simulink model "eVTOL_HIL"  (R2024b)
settings: Solver=FixedStepAuto  StartTime=0.0  StopTime=inf  FixedStep=SAMPLE_TIME  RelTol=1e-3
values from neighbouring files (symbols this model uses):
  aDl =     [initdata.mat]
  aDr =     [initdata.mat]
  aDyn =     [initdata.mat]
  aLat =     [initdata.mat]
  aLon =     [initdata.mat]
  D = Prop.D    [EOM_dt_MC.m]    (also in EOM_get_alf_dt_de_prop_evtol.m = CD * QS)
  General = init_layoutdata    [EOM_dt_MC.m]    (also in build_optimized_CA.m; initdata.mat = ; initdata_HIL_eVTOL.m)
  mass = Con(3)    [EOM_get_alf_dt_de_prop_evtol.m]    (also in initdata.mat = 2255.54; initdata_HIL_eVTOL.m = 7)
  Motor = init_motor_evtol    [EOM_dt_MC.m]    (also in initdata.mat = []; initdata_HIL_eVTOL.m)
  Prop = init_propeller_evtol_new    [EOM_dt_MC.m]    (also in initdata_HIL_eVTOL.m)
  SAMPLE_TIME = 0.01    [initdata_HIL_eVTOL.m]
undefined symbols (not defined in the file or in its folder): aDa, aDe, asbhl20env, Environment, InitData, magnitude
libraries: simulink_extras x16, vrlib x8, matrix_library x6, sharedutil x6, aerolibwindfilters x4, sharedtransform x4, aerolibfltsims x3, instrumentseriallib x3, uavmavlinklib x3, aerolibasang x3, aerolibobsolete x2, aerolibanimutils x1
(part 1 of 4)
settings Model: SimulationMode=accelerator  Creator=Administrator  LastModifiedBy=ZDB
settings DebuggingCC: UnderspecifiedInitializationDetection=Classic  MergeDetectMultiDrivingBlocksExec=none
settings ModelReferenceCC: PropagateSignalLabelsOutOfModel=off

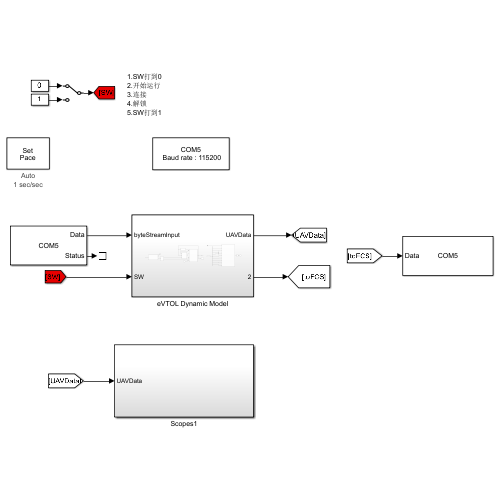
[thumbnail: Simulink's stored preview of the top-level diagram]
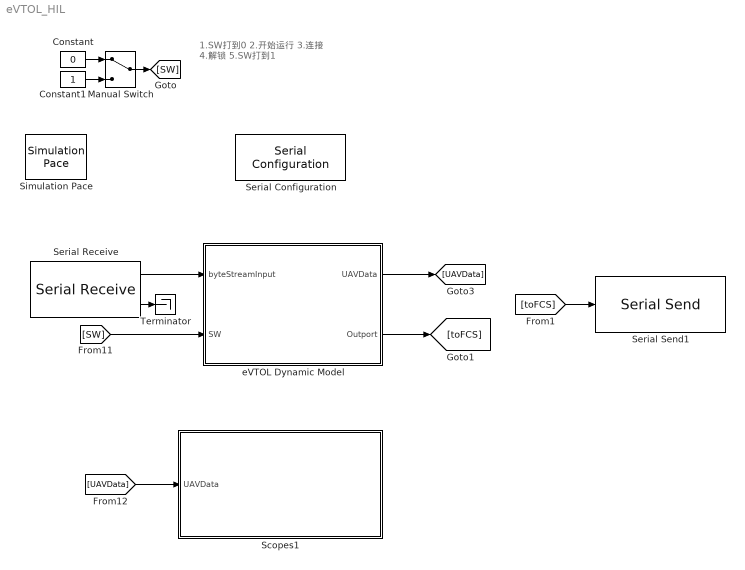
== system eVTOL_HIL ==
  note: 1.SW打到0
      | 2.开始运行
      | 3.连接
      | 4.解锁
      | 5.SW打到1
  Constant : Constant  Value=0
  Constant1 : Constant
  Manual Switch : ManualSwitch
  Scopes1 : Subsystem
  Serial Configuration : instrumentseriallib/Serial Configuration  Priority=-200000  PortSel=COM5  Port=COM5  ComPort=COM5  BaudRate=115200  DataBits=8  Parity=none  StopBits=1  ByteOrder=little-endian  FlowControl=none  Timeout=10  SimulateUsing=Interpreted execution  BlockInModel=on  aMode=1
  Serial Receive : instrumentseriallib/Serial Receive  PortSel=COM5  Port=COM5  ComPort=COM5  DataType=uint8  SaveDataType=uint8  ToggleHeader=off  Header=[253 37]  ToggleDataSize=on  DataSize=[49]  ToggleTerminator=off  Terminator=<none>  CustomTerminator=[]  InputFormat=Column major  EnableBlockingMode=off  ActionDataUnavailable=Output last received value  ActionWhenDataUnavailable=Output last received value  CustomValue=0  SampleTime=SAMPLE_TIME  SimulateUsing=Interpreted execution  BlockInModel=on  aMode=1
  Serial Send1 : instrumentseriallib/Serial Send  Priority=1  PortSel=COM5  Port=COM5  ComPort=COM5  Header=[]  Terminator=<none>  CustomTerminator=[]  EnableBlockingMode=off  SimulateUsing=Interpreted execution  BlockInModel=on  aMode=1
  Simulation Pace : aerolibanimutils/Simulation Pace  SimulationPace=1  SleepMode=Auto  OutputPaceError=off  SampleTime=-1
  Terminator : Terminator
  eVTOL Dynamic Model : Subsystem
  wires:
  Constant/1 -> Manual Switch/1
  Manual Switch/1 -> [SW]
  Constant1/1 -> Manual Switch/2
  Serial Receive/2 -> Terminator/1
  Serial Receive/1 -> eVTOL Dynamic Model/1(byteStreamInput)
  [SW] -> eVTOL Dynamic Model/2(SW)
  eVTOL Dynamic Model/1(UAVData) -> [UAVData]
  [toFCS] -> Serial Send1/1
  eVTOL Dynamic Model/2(Outport) -> [toFCS]
  [UAVData] -> Scopes1/1(UAVData)

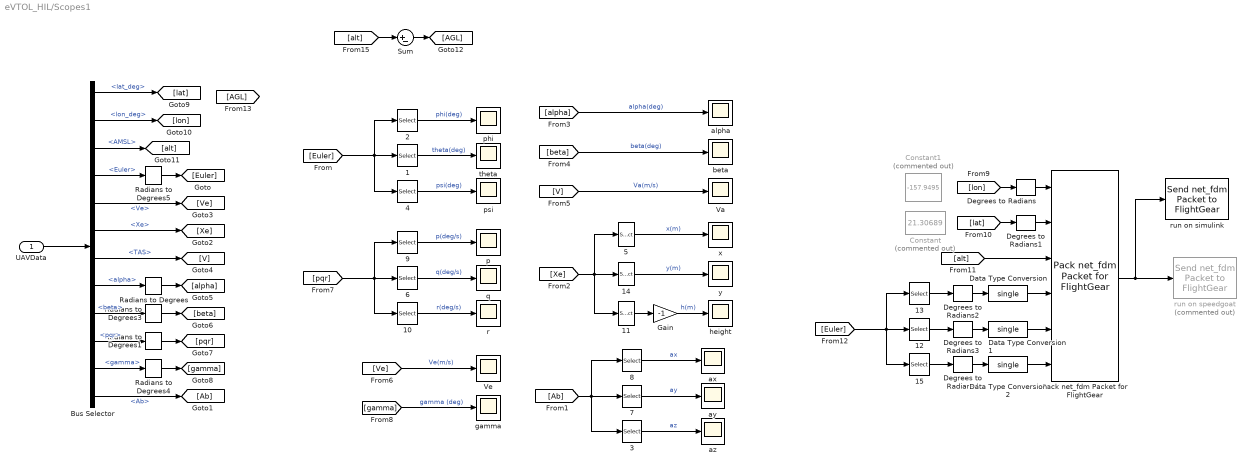
== system eVTOL_HIL/Scopes1 ==
  UAVData : Inport
  {1,6..7,12,14} (5 alike) : Selector  InputPortWidth=3  IndexOptions=Index vector (dialog)  Indices=2  OutputSizes=1
  {3..4,10..11,15} (5 alike) : Selector  InputPortWidth=3  IndexOptions=Index vector (dialog)  Indices=3  OutputSizes=1
  {2,5,8..9,13} (5 alike) : Selector  InputPortWidth=3  IndexOptions=Index vector (dialog)  Indices=1  OutputSizes=1
  Bus Selector : BusSelector  OutputSignals=lat_deg,lon_deg,AMSL,Euler,Ve,Xe,TAS,alpha,beta,pqr,gamma,Ab
  Constant : Constant  Commented=on  Value=21.30689
  Constant1 : Constant  Commented=on  Value=-157.9495
  Data Type Conversion : DataTypeConversion  OutDataTypeStr=single  SaturateOnIntegerOverflow=off  RndMeth=Floor
  Data Type Conversion1 : DataTypeConversion  OutDataTypeStr=single  SaturateOnIntegerOverflow=off  RndMeth=Floor
  Data Type Conversion2 : DataTypeConversion  OutDataTypeStr=single  SaturateOnIntegerOverflow=off  RndMeth=Floor
  Degrees to Radians{,1..4} (5 alike) : simulink_extras/Transformations/Degrees to Radians
  Gain : Gain  Gain=-1
  Pack net_fdm Packet for FlightGear : aerolibfltsims/Pack net_fdm Packet for FlightGear  FlightGearVersion=v2019.1  ShowPositionAttitudeInputs=on  ShowVelocityAccelerationInputs=off  ShowControlSurfacePositionInputs=off  ShowEngineFuelInputs=off  ShowLandingGearInputs=off  ShowEnvironmentInputs=off  SampleTime=-1  packetVersion=24
  Radians to Degrees{,1,3..5} (5 alike) : simulink_extras/Transformations/Radians to Degrees
  Sum : Sum  Inputs=|+-
  Va : Scope
  Ve : Scope
  alpha : Scope
  ax : Scope
  ay : Scope
  az : Scope
  beta : Scope
  gamma : Scope
  height : Scope
  p : Scope
  phi : Scope
  psi : Scope
  q : Scope
  r : Scope
  run on simulink : aerolibfltsims/Send net_fdm Packet to FlightGear  DestinationIpAddress=127.0.0.1  DestinationPort=5502  LocalIpPort=-1  varLen=off  SampleTime=0.01
  run on speedgoat : aerolibfltsims/Send net_fdm Packet to FlightGear  Commented=on  DestinationIpAddress=192.168.7.2  DestinationPort=5502  LocalIpPort=-1  varLen=off  SampleTime=-1
  theta : Scope
  x : Scope
  y : Scope
  wires:
  Radians to Degrees5/1 -> [Euler]
  UAVData/1 -> Bus Selector/1
  1/1 -> theta/1  "theta(deg)"
  Bus Selector/6 -> [Xe]  "<Xe>"
  2/1 -> phi/1  "phi(deg)"
  4/1 -> psi/1  "psi(deg)"
  Bus Selector/8 -> Radians to Degrees/1  "<alpha>"
  [Euler] -> 1/1, 2/1, 4/1
  Bus Selector/4 -> Radians to Degrees5/1  "<Euler>"
  [Xe] -> 5/1, 14/1, 11/1
  Bus Selector/5 -> [Ve]  "<Ve>"
  Bus Selector/7 -> [V]  "<TAS>"
  Radians to Degrees/1 -> [alpha]
  Bus Selector/9 -> Radians to Degrees3/1  "<beta>"
  Radians to Degrees3/1 -> [beta]
  [beta] -> beta/1  "beta(deg)"
  [alpha] -> alpha/1  "alpha(deg)"
  [Ve] -> Ve/1  "Ve(m/s)"
  Bus Selector/10 -> Radians to Degrees1/1  "<pqr>"
  6/1 -> q/1  "q(deg/s)"
  9/1 -> p/1  "p(deg/s)"
  10/1 -> r/1  "r(deg/s)"
  [pqr] -> 10/1, 9/1, 6/1
  Radians to Degrees1/1 -> [pqr]
  11/1 -> Gain/1
  Gain/1 -> height/1  "h(m)"
  5/1 -> x/1  "x(m)"
  Bus Selector/11 -> Radians to Degrees4/1  "<gamma>"
  Radians to Degrees4/1 -> [gamma]
  [gamma] -> gamma/1  "gamma (deg)"
  14/1 -> y/1  "y(m)"
  [V] -> Va/1  "Va(m/s)"
  Bus Selector/12 -> [Ab]  "<Ab>"
  [Ab] -> 8/1, 7/1, 3/1
  3/1 -> az/1  "az"
  8/1 -> ax/1  "ax"
  7/1 -> ay/1  "ay"
  Bus Selector/1 -> [lat]  "<lat_deg>"
  Bus Selector/2 -> [lon]  "<lon_deg>"
  Bus Selector/3 -> [alt]  "<AMSL>"
  Pack net_fdm Packet for FlightGear/1 -> run on simulink/1, run on speedgoat/1
  Degrees to Radians1/1 -> Pack net_fdm Packet for FlightGear/2
  Data Type Conversion/1 -> Pack net_fdm Packet for FlightGear/4
  Degrees to Radians/1 -> Pack net_fdm Packet for FlightGear/1
  12/1 -> Degrees to Radians3/1
  Data Type Conversion1/1 -> Pack net_fdm Packet for FlightGear/5
  13/1 -> Degrees to Radians2/1
  15/1 -> Degrees to Radians4/1
  Data Type Conversion2/1 -> Pack net_fdm Packet for FlightGear/6
  [alt] -> Pack net_fdm Packet for FlightGear/3
  Degrees to Radians2/1 -> Data Type Conversion/1
  Degrees to Radians3/1 -> Data Type Conversion1/1
  Degrees to Radians4/1 -> Data Type Conversion2/1
  [lon] -> Degrees to Radians/1
  [lat] -> Degrees to Radians1/1
  [Euler] -> 15/1, 13/1, 12/1
  Sum/1 -> [AGL]
  [alt] -> Sum/1

== system eVTOL_HIL/eVTOL Dynamic Model ==
  byteStreamInput : Inport
  SW : Inport  Port=2
  Bus Selector : BusSelector  OutputSignals=DCM_be,pqr,lat_deg,lon_deg,AMSL,Ve,Ab,EAS,TAS
  Clock1 : Clock
  Energy & Power : Subsystem
  Environment : Subsystem  AncestorBlock=asbhl20env/Environment  TreatAsAtomicUnit=on
      settings: LibrarySourceBlock=asbhl20env/Environment
  MAVLink Deserializer1 : uavmavlinklib/MAVLink Deserializer  dialectSource=Select from standard MAVLink dialects  dialect=common.xml  dialectCustom=common.xml  version=2  messageType=SERVO_OUTPUT_RAW  inputDataLength=off  SystemIDFilter=off  systemID=1  ComponentIDFilter=off  componentID=1  queueMsg=off  queueMsgSize=50  dropNum=off
  Mux : Mux  Inputs=2
  Rate Transition : RateTransition  OutPortSampleTime=0.01
  Scope1 : Scope
  airframe : Subsystem
  hil_state_quaternion_pack1 : Subsystem
  信号处理 : Subsystem
  UAVData : Outport
  Outport : Outport  Port=2
  wires:
  MAVLink Deserializer1/1 -> Scope1/1  "status"
  byteStreamInput/1 -> MAVLink Deserializer1/1
  MAVLink Deserializer1/2 -> 信号处理/1(Msg)
  SW/1 -> airframe/4(SW)
  信号处理/2(Act_surface) -> airframe/3(Act_surface)
  Energy & Power/1(PropData) -> airframe/2(prop)
  Environment/1(Envm) -> Energy & Power/1(EnvData), airframe/1(EnvmData)
  信号处理/1(Act_T) -> Energy & Power/3(Act_T)
  Bus Selector/9 -> hil_state_quaternion_pack1/9(TAS)  "<TAS>"
  Rate Transition/1 -> Outport/1
  Bus Selector/4 -> Mux/2  "<lon_deg>"
  Bus Selector/5 -> hil_state_quaternion_pack1/5(amsl)  "<AMSL>"
  Bus Selector/6 -> hil_state_quaternion_pack1/6(Ve)  "<Ve>"
  Bus Selector/3 -> Mux/1  "<lat_deg>"
  Clock1/1 -> hil_state_quaternion_pack1/1(time_s)  "time_s"
  Bus Selector/7 -> hil_state_quaternion_pack1/7(ab)  "<Ab>"
  Bus Selector/1 -> hil_state_quaternion_pack1/2(DCM_be)  "<DCM_be>"
  Bus Selector/8 -> hil_state_quaternion_pack1/8(EAS)  "<EAS>"
  Mux/1 -> hil_state_quaternion_pack1/4(latlon_deg)
  hil_state_quaternion_pack1/1(Data to px4) -> Rate Transition/1
  [UAVData] -> Bus Selector/1
  Bus Selector/2 -> hil_state_quaternion_pack1/3(body_rate)  "<pqr>"
  airframe/1(UAVData) -> [UAVData], UAVData/1, Environment/1(plane), Energy & Power/2(UAVData)

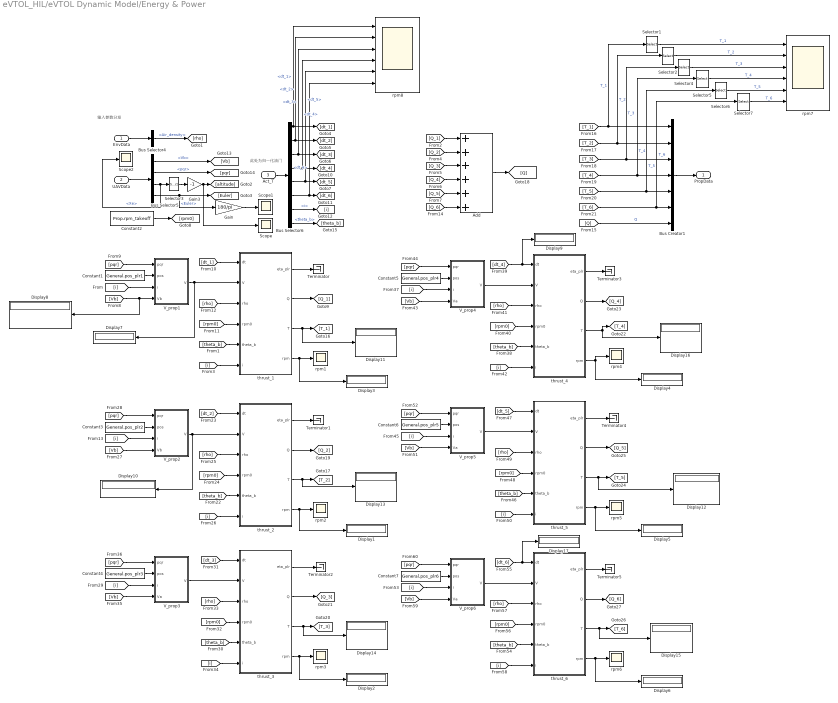
== system eVTOL_HIL/eVTOL Dynamic Model/Energy & Power ==
  note: 此处为归一化油门
  note: 输入参数分发
  EnvData : Inport
  UAVData : Inport  Port=2
  Act_T : Inport  Port=3
  Add : Sum  Inputs=++++++
  Bus Creator1 : BusCreator  Inputs=7
  Bus Selector4 : BusSelector  OutputSignals=Air_density
  Bus Selector5 : BusSelector  OutputSignals=Vb,pqr,Xe,Euler
  Bus Selector6 : BusSelector  OutputSignals=dt_1,dt_2,dt_3,dt_4,dt_5,dt_6,i,theta_b
  Constant1 : Constant  Value=General.pos_plr1
  Constant2 : Constant  Value=Prop.rpm_takeoff
  Constant3 : Constant  Value=General.pos_plr2
  Constant4 : Constant  Value=General.pos_plr3
  Constant5 : Constant  Value=General.pos_plr4
  Constant6 : Constant  Value=General.pos_plr5
  Constant7 : Constant  Value=General.pos_plr6
  Display{1..17} (17 alike) : Display
  Gain : Gain  Gain=180/pi
  Gain3 : Gain  Gain=-1
  Scope : Scope
  Scope1 : Scope
  Scope2 : Scope
  Selector{1..7} (7 alike) : Selector  InputPortWidth=3  IndexOptions=Index vector (dialog)  Indices=3  OutputSizes=1
  Terminator{,1..5} (6 alike) : Terminator
  V_prop1 : Subsystem
  V_prop2 : Subsystem
  V_prop3 : Subsystem
  V_prop4 : Subsystem
  V_prop5 : Subsystem
  V_prop6 : Subsystem
  rpm{1..6} (6 alike) : Scope
  rpm7 : Scope  NumInputPorts=6
  rpm8 : Scope  NumInputPorts=6
  thrust_1 : Subsystem
  thrust_2 : Subsystem
  thrust_3 : Subsystem
  thrust_4 : Subsystem
  thrust_5 : Subsystem
  thrust_6 : Subsystem
  PropData : Outport  VectorParamsAs1DForOutWhenUnconnected=off
  wires:
  Act_T/1 -> Bus Selector6/1
  [dt_1] -> thrust_1/1(dt)
  thrust_1/4(rpm) -> Display3/1, rpm1/1
  Constant1/1 -> V_prop1/2(pos)
  [rho] -> thrust_1/3(rho)
  [rpm0] -> thrust_1/4(rpm0)
  thrust_1/1(eta_plr) -> Terminator/1
  [pqr] -> V_prop1/1(pqr)
  [Vb] -> Display8/1, V_prop1/4(Vb)
  EnvData/1 -> Bus Selector4/1
  Bus Selector4/1 -> [rho]  "<Air_density>"
  Bus Selector5/2 -> [pqr]  "<pqr>"
  Selector3/1 -> Gain3/1
  UAVData/1 -> Bus Selector5/1
  Bus Selector5/4 -> Gain/1, [Euler]  "<Euler>"
  Bus Selector5/1 -> [Vb]  "<Vb>"
  Bus Selector5/3 -> Scope2/1, Selector3/1  "<Xe>"
  Bus Selector6/1 -> rpm8/1, [dt_1]  "<dt_1>"
  Bus Selector6/5 -> [dt_5], rpm8/5  "<dt_5>"
  Bus Selector6/3 -> [dt_3], rpm8/3  "<dt_3>"
  Bus Selector6/2 -> [dt_2], rpm8/2  "<dt_2>"
  V_prop1/1(V) -> thrust_1/2(V), Display7/1
  [i] -> V_prop1/3(i)
  Constant2/1 -> [rpm0]
  [theta_b] -> thrust_1/5(theta_b)
  thrust_1/2(Q) -> [Q_1]
  Bus Selector6/4 -> [dt_4], rpm8/4  "<dt_4>"
  Bus Selector6/6 -> rpm8/6, [dt_6]  "<dt_6>"
  Bus Selector6/7 -> [i]  "<i>"
  Bus Selector6/8 -> [theta_b]  "<theta_b>"
  [i] -> thrust_1/6(i)
  thrust_1/3(T) -> Display11/1, [T_1]
  [Q_1] -> Add/1
  [Q_6] -> Add/6
  [Q_5] -> Add/5
  [Q_4] -> Add/4
  [Q_3] -> Add/3
  [Q_2] -> Add/2
  Add/1 -> [Q]
  [Q] -> Bus Creator1/7  "Q"
  [T_1] -> Selector1/1, Bus Creator1/1  "T_1"
  [T_2] -> Selector2/1, Bus Creator1/2  "T_2"
  [T_3] -> Bus Creator1/3, Selector4/1  "T_3"
  [T_4] -> Bus Creator1/4, Selector5/1  "T_4"
  [T_5] -> Bus Creator1/5, Selector6/1  "T_5"
  [T_6] -> Bus Creator1/6, Selector7/1  "T_6"
  Bus Creator1/1 -> PropData/1
  [theta_b] -> thrust_2/5(theta_b)
  Constant3/1 -> V_prop2/2(pos)
  [dt_2] -> thrust_2/1(dt)
  V_prop2/1(V) -> Display10/1, thrust_2/2(V)
  thrust_2/2(Q) -> [Q_2]
  thrust_2/1(eta_plr) -> Terminator1/1
  [i] -> V_prop2/3(i)
  thrust_2/3(T) -> [T_2], Display13/1
  [rpm0] -> thrust_2/4(rpm0)
  [Vb] -> V_prop2/4(Vb)
  [pqr] -> V_prop2/1(pqr)
  [i] -> thrust_2/6(i)
  thrust_2/4(rpm) -> rpm2/1, Display1/1
  [rho] -> thrust_2/3(rho)
  [rho] -> thrust_3/3(rho)
  [pqr] -> V_prop3/1(pqr)
  [Vb] -> V_prop3/4(Va)
  [i] -> V_prop3/3(i)
  thrust_3/2(Q) -> [Q_3]
  V_prop3/1(V) -> thrust_3/2(V)
  [rpm0] -> thrust_3/4(rpm0)
  [dt_3] -> thrust_3/1(dt)
  thrust_3/4(rpm) -> Display2/1, rpm3/1
  [theta_b] -> thrust_3/5(theta_b)
  Constant4/1 -> V_prop3/2(pos)
  thrust_3/1(eta_plr) -> Terminator2/1
  [i] -> thrust_3/6(i)
  thrust_3/3(T) -> Display14/1, [T_3]
  [i] -> thrust_4/6(i)
  [theta_b] -> thrust_4/5(theta_b)
  Constant5/1 -> V_prop4/2(pos)
  thrust_4/1(eta_plr) -> Terminator3/1
  thrust_4/3(T) -> [T_4], Display16/1
  [dt_4] -> Display9/1, thrust_4/1(dt)
  V_prop4/1(V) -> thrust_4/2(V)
  [rpm0] -> thrust_4/4(rpm0)
  [i] -> V_prop4/3(i)
  thrust_4/4(rpm) -> rpm4/1, Display4/1
  [Vb] -> V_prop4/4(Va)
  [pqr] -> V_prop4/1(pqr)
  [rho] -> thrust_4/3(rho)
  thrust_4/2(Q) -> [Q_4]
  thrust_5/2(Q) -> [Q_5]
  thrust_5/3(T) -> Display12/1, [T_5]
  [rho] -> thrust_5/3(rho)
  [pqr] -> V_prop5/1(pqr)
  [rpm0] -> thrust_5/4(rpm0)
  Constant6/1 -> V_prop5/2(pos)
  thrust_5/1(eta_plr) -> Terminator4/1
  [dt_5] -> thrust_5/1(dt)
  thrust_5/4(rpm) -> Display5/1, rpm5/1
  [i] -> V_prop5/3(i)
  V_prop5/1(V) -> thrust_5/2(V)
  [i] -> thrust_5/6(i)
  [theta_b] -> thrust_5/5(theta_b)
  [Vb] -> V_prop5/4(Va)
  [i] -> V_prop6/3(i)
  [Vb] -> V_prop6/4(Va)
  thrust_6/1(eta_plr) -> Terminator5/1
  V_prop6/1(V) -> thrust_6/2(V)
  [dt_6] -> Display17/1, thrust_6/1(dt)
  [theta_b] -> thrust_6/5(theta_b)
  thrust_6/2(Q) -> [Q_6]
  thrust_6/3(T) -> Display15/1, [T_6]
  Constant7/1 -> V_prop6/2(pos)
  [rho] -> thrust_6/3(rho)
  thrust_6/4(rpm) -> Display6/1, rpm6/1
  [pqr] -> V_prop6/1(pqr)
  [rpm0] -> thrust_6/4(rpm0)
  [i] -> thrust_6/6(i)
  Selector1/1 -> rpm7/1  "T_1"
  Selector2/1 -> rpm7/2  "T_2"
  Selector4/1 -> rpm7/3  "T_3"
  Selector5/1 -> rpm7/4  "T_4"
  Selector6/1 -> rpm7/5  "T_5"
  Selector7/1 -> rpm7/6  "T_6"
  Gain3/1 -> Scope/1, [altitude]
  Gain/1 -> Scope1/1

== system eVTOL_HIL/eVTOL Dynamic Model/Environment ==
  plane : Inport
  Bus Creator : BusCreator  Inputs=8
  Bus Selector : BusSelector  OutputSignals=Xe,Ve,DCM_be
  COESA Atmosphere Model : aerolibatmos2/COESA Atmosphere Model  units=Metric (MKS)  spec=1976 COESA-extended U.S. Standard Atmosphere  model=Profile  profile_var=High temperature  profile_percent=1%  profile_alt=5 km (16404 ft)  envelope_var=High temperature  envelope_percent=1%  action=Warning
  Height : Selector  InputPortWidth=3  IndexOptions=Index vector (dialog)  Indices=[3]  OutputSizes=1
  Latitude : Constant  Value=40
  Terrain : Subsystem
  WGS84 Gravity Model : aerolibobsolete/WGS84 Gravity Model  model=WGS84 Taylor Series  units=Metric (MKS)  no_atmos=on  precessing=on  month=February  day=1  year=2000  no_centrifugal=on  action=None
  Wind Models : Subsystem
  x : Selector  InputPortWidth=3  IndexOptions=Index vector (dialog)  Indices=1  OutputSizes=1
  z-->h : Abs
  Envm : Outport  InitialOutput=0  VectorParamsAs1DForOutWhenUnconnected=off
  wires:
  Bus Selector/1 -> x/1, Terrain/1(Xe), Height/1  "<Xe>"
  Bus Selector/3 -> Wind Models/4(DCM)  "<DCM_be>"
  Wind Models/1(ug,vg,wg1) -> Bus Creator/2  "WindVelocity"
  Height/1 -> z-->h/1
  Latitude/1 -> WGS84 Gravity Model/2
  Wind Models/2(pg,qg,rg1) -> Bus Creator/3  "WindAngularRate"
  Bus Creator/1 -> Envm/1  "EnvmData"
  z-->h/1 -> COESA Atmosphere Model/1, WGS84 Gravity Model/1, Wind Models/3(Altitude)
  COESA Atmosphere Model/2 -> Bus Creator/5  "a"
  plane/1 -> Bus Selector/1
  COESA Atmosphere Model/3 -> Bus Creator/6  "Air_pressure"
  Bus Selector/2 -> Wind Models/2(Ve)  "<Ve>"
  COESA Atmosphere Model/4 -> Bus Creator/7  "Air_density"
  x/1 -> Wind Models/1(Xe_x)
  COESA Atmosphere Model/1 -> Bus Creator/4  "T(K)"
  Terrain/1(hground) -> Bus Creator/1  "hground"
  WGS84 Gravity Model/1 -> Bus Creator/8  "g"

== system eVTOL_HIL/eVTOL Dynamic Model/airframe ==
  EnvmData : Inport
  prop : Inport  Port=2
  Act_surface : Inport  Port=3
  SW : Inport  Port=4
  6DoF (Euler Angles)1 : aerolibobsolete/6DoF (Euler Angles)  units=Metric (MKS)  mtype=Fixed  rep=Euler Angles  xme_0=InitData.Xe  Vm_0=InitData.Vb  eul_0=InitData.Euler+[0,0,0]/57.3  pm_0=InitData.pqr  mass_0=InitData.mass0  mass_e=0.5  mass_f=2.0  inertia=Mass.Inertial  inertia_e=eye(3)  inertia_f=2*eye(3)  k_quat=1.0
  Bus Creator : BusCreator  Inputs=27
  Constant3 : Constant  Value=mass
  Flight Conditions : Subsystem  AncestorBlock=asbhl20vehicle/Vehicle/Aerodynamic/DerivedConditions
      settings: LibrarySourceBlock=asbhl20vehicle/Vehicle/Aerodynamic/DerivedConditions
  Fly : Constant
  Gain : Gain  Gain=[1,1,1]
  Gain1 : Gain  Gain=[1,1,1]
  Product : Product
  Product1 : Product
  Radians to Degrees{1..4,7..8} (6 alike) : simulink_extras/Transformations/Radians to Degrees
  Selector1 : Selector  InputPortWidth=3  IndexOptions=Index vector (dialog)  Indices=[2]  OutputSizes=1
  Selector2 : Selector  InputPortWidth=3  IndexOptions=Index vector (dialog)  Indices=[2]  OutputSizes=1
  Selector3 : Selector  InputPortWidth=3  IndexOptions=Index vector (dialog)  Indices=[1]  OutputSizes=1
  Selector4 : Selector  InputPortWidth=3  IndexOptions=Index vector (dialog)  Indices=[3]  OutputSizes=1
  Selector5 : Selector  InputPortWidth=3  IndexOptions=Index vector (dialog)  Indices=[1]  OutputSizes=1
  Selector6 : Selector  InputPortWidth=3  IndexOptions=Index vector (dialog)  Indices=[3]  OutputSizes=1
  Switch2 : Switch  Criteria=u2 > Threshold  SaturateOnIntegerOverflow=off  InputSameDT=off
  force moment : Subsystem
  fw_phi : Scope
  fw_psi : Scope
  fw_theta : Scope
  init : Constant  Value=0
  p : Scope
  q : Scope
  r : Scope
  UAVData : Outport  VectorParamsAs1DForOutWhenUnconnected=off
  wires:
  prop/1 -> force moment/3(prop)
  6DoF (Euler Angles)1/1 -> Bus Creator/1  "Ve"
  6DoF (Euler Angles)1/2 -> Bus Creator/2  "Xe"
  6DoF (Euler Angles)1/8 -> Bus Creator/8  "Ab"
  6DoF (Euler Angles)1/7 -> Bus Creator/7  "pqr_dot"
  6DoF (Euler Angles)1/5 -> Bus Creator/5  "Vb"
  Act_surface/1 -> force moment/2(Act_surface)
  Bus Creator/1 -> UAVData/1, force moment/1(PlantData), Flight Conditions/2(UAVData)  "UAVData"
  EnvmData/1 -> Flight Conditions/1(EnvData), force moment/4(EnvmData)
  6DoF (Euler Angles)1/4 -> Bus Creator/4  "DCM_be"
  Constant3/1 -> Bus Creator/23  "mass"
  force moment/1(Fb (X Y Z)) -> Gain/1
  force moment/2(M (L M N)) -> Gain1/1
  Product/1 -> 6DoF (Euler Angles)1/1
  Gain1/1 -> Product1/2
  Product1/1 -> 6DoF (Euler Angles)1/2
  Gain/1 -> Product/2
  Fly/1 -> Switch2/1
  init/1 -> Switch2/3
  Switch2/1 -> Product1/1, Product/1  "是否关闭力输出"
  SW/1 -> Switch2/2
  Flight Conditions/1(lat_deg) -> Bus Creator/9
  Flight Conditions/2(lon_deg) -> Bus Creator/10
  Flight Conditions/3(AMSL) -> Bus Creator/11
  Flight Conditions/4(gamma) -> Bus Creator/12
  Flight Conditions/5(chi) -> Bus Creator/13
  Flight Conditions/6(alphaDot) -> Bus Creator/14
  Flight Conditions/7(alpha) -> Bus Creator/15
  Flight Conditions/8(beta) -> Bus Creator/16
  Flight Conditions/9(TAS) -> Bus Creator/17
  Flight Conditions/10(pqr_air) -> Bus Creator/18
  Flight Conditions/11(Mach) -> Bus Creator/19  "mach"
  Flight Conditions/12(DynamicPressure) -> Bus Creator/20
  Flight Conditions/13(EAS) -> Bus Creator/21
  Flight Conditions/14(T(K)) -> Bus Creator/22
  Flight Conditions/15(Air_pressure) -> Bus Creator/24
  Flight Conditions/16(g) -> Bus Creator/25
  Flight Conditions/17(Vb_air) -> Bus Creator/26  "Va"
  Flight Conditions/18(Ve_Inertial) -> Bus Creator/27
  Radians to Degrees2/1 -> fw_psi/1
  Selector4/1 -> Radians to Degrees2/1
  Radians to Degrees3/1 -> fw_phi/1
  Radians to Degrees1/1 -> fw_theta/1
  6DoF (Euler Angles)1/3 -> Bus Creator/3, Selector2/1, Selector3/1, Selector4/1  "Euler"
  Selector3/1 -> Radians to Degrees3/1
  Selector2/1 -> Radians to Degrees1/1
  Radians to Degrees7/1 -> r/1
  Selector6/1 -> Radians to Degrees7/1
  Selector5/1 -> Radians to Degrees8/1
  Radians to Degrees4/1 -> q/1
  Selector1/1 -> Radians to Degrees4/1
  Radians to Degrees8/1 -> p/1
  6DoF (Euler Angles)1/6 -> Selector6/1, Selector5/1, Selector1/1, Bus Creator/6  "pqr"

== system eVTOL_HIL/eVTOL Dynamic Model/hil_state_quaternion_pack1 ==
  time_s : Inport
  DCM_be : Inport  Port=2
  body_rate : Inport  Port=3
  latlon_deg : Inport  Port=4
  amsl : Inport  Port=5
  Ve : Inport  Port=6
  ab : Inport  Port=7
  EAS : Inport  Port=8
  TAS : Inport  Port=9
  Bus Assignment : BusAssignment  AssignedSignals=signal1
  Bus Creator : BusCreator  Inputs=5  OutDataTypeStr=Bus: SL_Bus_MAVLink_HIL_STATE_QUATERNION_Packet  NonVirtualBus=on
  Bus Selector : BusSelector  OutputSignals=MsgID,SystemID,ComponentID,Sequence
  MAVLink Blank Message2 : uavmavlinklib/MAVLink Blank Message  dialectSource=Select from standard MAVLink dialects  dialect=common.xml  dialectCustom=common.xml  version=2  messageType=HIL_STATE_QUATERNION  SystemID=SYS_ID  ComponentID=COMP_ID  SampleTime=SAMPLE_TIME
  MAVLink Serializer2 : uavmavlinklib/MAVLink Serializer  dialectSource=Select from standard MAVLink dialects  dialect=common.xml  dialectCustom=common.xml  version=2  messageType=HIL_STATE_QUATERNION
  Signal Conversion : SignalConversion  ConversionOutput=Nonvirtual bus  OverrideOpt=off
  Terminator2 : Terminator
  payload_hil_state_quaternion : Subsystem
  Data to px4 : Outport
  wires:
  Signal Conversion/1 -> MAVLink Serializer2/1
  Bus Creator/1 -> Signal Conversion/1
  EAS/1 -> payload_hil_state_quaternion/8(EAS)
  ab/1 -> payload_hil_state_quaternion/7(ab)
  TAS/1 -> payload_hil_state_quaternion/9(TAS)
  Ve/1 -> payload_hil_state_quaternion/6(Ve)
  DCM_be/1 -> payload_hil_state_quaternion/2(DCM_be)
  amsl/1 -> payload_hil_state_quaternion/5(amsl)
  body_rate/1 -> payload_hil_state_quaternion/3(body_rate)
  time_s/1 -> payload_hil_state_quaternion/1(time_s)
  Bus Selector/1 -> Bus Creator/1  "<MsgID>"
  Bus Selector/2 -> Bus Creator/2  "<SystemID>"
  Bus Selector/4 -> Bus Creator/4  "<Sequence>"
  Bus Selector/3 -> Bus Creator/3  "<ComponentID>"
  payload_hil_state_quaternion/1(Payload) -> Bus Creator/5
  MAVLink Blank Message2/1 -> Bus Selector/1
  MAVLink Serializer2/1 -> Data to px4/1  "status"
  MAVLink Serializer2/2 -> Terminator2/1
  latlon_deg/1 -> payload_hil_state_quaternion/4(latlon_deg)

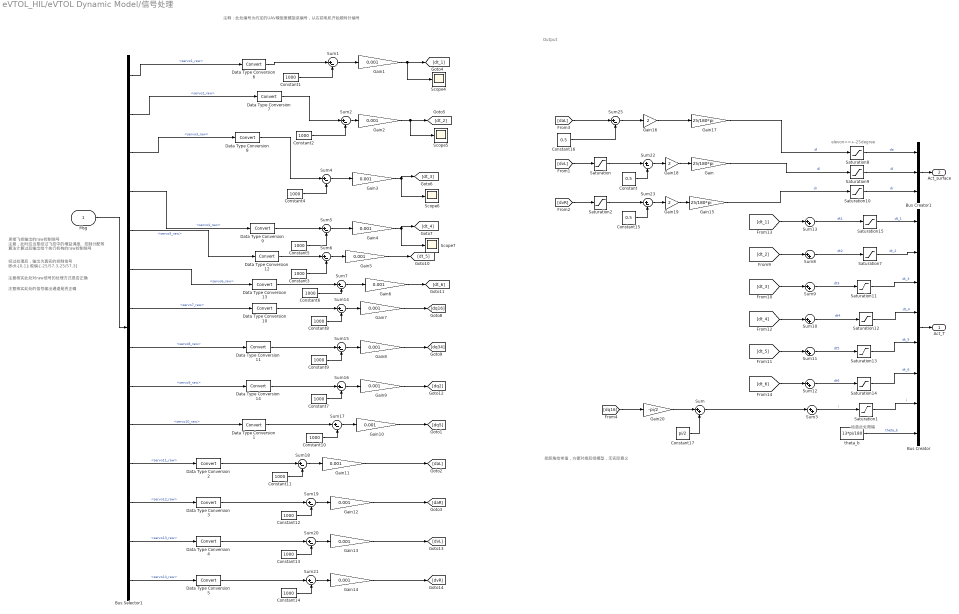
== system eVTOL_HIL/eVTOL Dynamic Model/信号处理 ==
  note: 桨距角给常值，方便对接后续模型，无实际意义
  note: 检查此处限幅
  note: 注意核实此处的信号输出通道是否正确
  note: 经过处理后，输出为真实的控制信号
      | 即dt-[0,1]; 舵偏-[-25/57.3,25/57.3]
  note: 注意核实此处对raw信号的处理方式是否正确
  note: 承接飞控输出的raw控制信号
      | 注意，此时应当是经过飞控中的增益调度、控制分配等
      | 算法计算过后输出给个执行机构的raw控制信号
  note: 注释：此处编号为约定的UAV模型里螺旋桨编号，从右前电机开始顺时针编号
  note: Output
  note: elevon==+-25degree
  Msg : Inport
  Bus Creator : BusCreator  Inputs=8
  Bus Creator1 : BusCreator  Inputs=3
  Bus Selector1 : BusSelector  OutputSignals=Payload.servo1_raw,Payload.servo2_raw,Payload.servo3_raw,Payload.servo4_raw,Payload.servo5_raw,Payload.servo6_raw,Payload.servo7_raw,Payload.servo8_raw,Payload.servo9_raw,Payload.servo10_raw,Payload.servo11_raw,Payload.servo12_raw,Payload.servo13_raw,Payload.servo14_raw
  Constant : Constant  Value=0.5
  Constant{1..14} (14 alike) : Constant  Value=1000
  Constant15 : Constant  Value=0.5
  Constant16 : Constant  Value=0.5
  Constant17 : Constant  Value=pi/2
  Data Type Conversion{1..14} (14 alike) : DataTypeConversion  SaturateOnIntegerOverflow=off  RndMeth=Floor
  Gain : Gain  Gain=25/180*pi
  Gain{1..14} (14 alike) : Gain  Gain=0.001
  Gain15 : Gain  Gain=25/180*pi
  Gain16 : Gain  Gain=2
  Gain17 : Gain  Gain=25/180*pi
  Gain18 : Gain  Gain=2
  Gain19 : Gain  Gain=2
  Gain20 : Gain  Gain=-pi/2
  Saturation{,2,7,11..15} (8 alike) : Saturate  UpperLimit=1  LowerLimit=0
  Saturation1 : Saturate  UpperLimit=90/57.3  LowerLimit=0
  Saturation10 : Saturate  UpperLimit=25/57.3  LowerLimit=-25/57.3
  Saturation8 : Saturate  UpperLimit=25/57.3  LowerLimit=-25/57.3
  Saturation9 : Saturate  UpperLimit=25/57.3  LowerLimit=-25/57.3
  Scope{4..7} (4 alike) : Scope
  Sum{,3,8..13} (8 alike) : Sum  Inputs=|++
  Sum{1..2,4..7,14..23,25} (17 alike) : Sum  Inputs=|+-
  theta_b : Constant  Value=13*pi/180
  Act_T : Outport
  Act_surface : Outport  Port=2
  wires:
  Saturation8/1 -> Bus Creator1/1  "da"
  Saturation9/1 -> Bus Creator1/2  "dl"
  Bus Creator1/1 -> Act_surface/1
  Data Type Conversion6/1 -> Sum1/1
  Gain1/1 -> [dt_1], Scope4/1
  Sum1/1 -> Gain1/1
  Constant1/1 -> Sum1/2
  Bus Selector1/1 -> Data Type Conversion6/1  "<servo1_raw>"
  Gain2/1 -> [dt_2], Scope5/1
  Constant2/1 -> Sum2/2
  Data Type Conversion7/1 -> Sum2/1
  Sum2/1 -> Gain2/1
  Bus Selector1/2 -> Data Type Conversion7/1  "<servo2_raw>"
  Gain3/1 -> [dt_3], Scope6/1
  Constant4/1 -> Sum4/2
  Data Type Conversion8/1 -> Sum4/1
  Sum4/1 -> Gain3/1
  Bus Selector1/3 -> Data Type Conversion8/1  "<servo3_raw>"
  Gain4/1 -> [dt_4], Scope7/1
  Constant5/1 -> Sum5/2
  Data Type Conversion9/1 -> Sum5/1
  Sum5/1 -> Gain4/1
  Bus Selector1/4 -> Data Type Conversion9/1  "<servo4_raw>"
  Gain7/1 -> [dq16]
  Data Type Conversion10/1 -> Sum14/1
  Gain/1 -> Saturation9/1  "dl"
  Msg/1 -> Bus Selector1/1
  Gain5/1 -> [dt_5]
  Sum6/1 -> Gain5/1
  Data Type Conversion12/1 -> Sum6/1
  Bus Selector1/5 -> Data Type Conversion12/1  "<servo5_raw>"
  Gain6/1 -> [dt_6]
  Sum7/1 -> Gain6/1
  Bus Selector1/6 -> Data Type Conversion13/1  "<servo6_raw>"
  Bus Selector1/7 -> Data Type Conversion10/1  "<servo7_raw>"
  Bus Selector1/8 -> Data Type Conversion11/1  "<servo8_raw>"
  Bus Selector1/9 -> Data Type Conversion14/1  "<servo9_raw>"
  Gain15/1 -> Saturation10/1  "dr"
  Saturation10/1 -> Bus Creator1/3  "dr"
  [dt_6] -> Sum12/1
  [dt_4] -> Sum10/1
  Saturation7/1 -> Bus Creator/2  "dt_2"
  [dt_5] -> Sum11/1
  [dt_3] -> Sum9/1
  Sum11/1 -> Saturation13/1  "dt5"
  Saturation13/1 -> Bus Creator/5  "dt_5"
  Saturation14/1 -> Bus Creator/6  "dt_6"
  Sum8/1 -> Saturation7/1  "dt2"
  Saturation15/1 -> Bus Creator/1  "dt_1"
  Sum12/1 -> Saturation14/1  "dt6"
  [dt_2] -> Sum8/1
  Sum9/1 -> Saturation11/1  "dt3"
  Sum10/1 -> Saturation12/1  "dt4"
  Sum13/1 -> Saturation15/1  "dt1"
  [dt_1] -> Sum13/1
  Saturation11/1 -> Bus Creator/3  "dt_3"
  Saturation12/1 -> Bus Creator/4  "dt_4"
  Gain10/1 -> [dq5]
  Bus Selector1/10 -> Data Type Conversion1/1  "<servo10_raw>"
  Bus Creator/1 -> Act_T/1
  Saturation1/1 -> Bus Creator/7  "i"
  Sum3/1 -> Saturation1/1  "i"
  Sum/1 -> Sum3/1
  theta_b/1 -> Bus Creator/8  "theta_b"
  Bus Selector1/11 -> Data Type Conversion2/1  "<servo11_raw>"
  Bus Selector1/12 -> Data Type Conversion3/1  "<servo12_raw>"
  Bus Selector1/13 -> Data Type Conversion4/1  "<servo13_raw>"
  Bus Selector1/14 -> Data Type Conversion5/1  "<servo14_raw>"
  Constant3/1 -> Sum6/2
  Data Type Conversion13/1 -> Sum7/1
  Constant6/1 -> Sum7/2
  Constant8/1 -> Sum14/2
  Sum14/1 -> Gain7/1
  Constant9/1 -> Sum15/2
  Sum15/1 -> Gain8/1
  Data Type Conversion11/1 -> Sum15/1
  Gain8/1 -> [dq34]
  Constant7/1 -> Sum16/2
  Sum16/1 -> Gain9/1
  Data Type Conversion14/1 -> Sum16/1
  Gain9/1 -> [dq2]
  Constant10/1 -> Sum17/2
  Sum17/1 -> Gain10/1
  Data Type Conversion1/1 -> Sum17/1
  Constant11/1 -> Sum18/2
  Sum18/1 -> Gain11/1
  Data Type Conversion2/1 -> Sum18/1
  Gain11/1 -> [daL]
  Constant12/1 -> Sum19/2
  Sum19/1 -> Gain12/1
  Data Type Conversion3/1 -> Sum19/1
  Constant13/1 -> Sum20/2
  Sum20/1 -> Gain13/1
  Data Type Conversion4/1 -> Sum20/1
  Constant14/1 -> Sum21/2
  Sum21/1 -> Gain14/1
  Data Type Conversion5/1 -> Sum21/1
  Gain14/1 -> [dvR]
  Gain13/1 -> [dvL]
  Gain12/1 -> [daR]
  Sum23/1 -> Gain19/1
  Saturation2/1 -> Sum23/1
  Sum22/1 -> Gain18/1
  Constant15/1 -> Sum23/2
  [dvL] -> Saturation/1
  Saturation/1 -> Sum22/1
  [dvR] -> Saturation2/1
  Constant/1 -> Sum22/2
  Sum25/1 -> Gain16/1
  [daL] -> Sum25/1
  Gain16/1 -> Gain17/1
  Constant16/1 -> Sum25/2
  Gain17/1 -> Saturation8/1  "dl"
  Gain18/1 -> Gain/1
  Gain19/1 -> Gain15/1
  [dq16] -> Gain20/1
  Gain20/1 -> Sum/1
  Constant17/1 -> Sum/2

== system eVTOL_HIL/eVTOL Dynamic Model/Energy & Power/V_prop1 ==
  note: 将速度矢量投影到桨轴
  pqr : Inport
  pos : Inport  Port=2
  i : Inport  Port=3
  Vb : Inport  Port=4
  Cross Product4 : matrix_library/Cross Product
  Display1 : Display
  Display2 : Display
  Display8 : Display
  Sum2 : Sum  Inputs=|++
  v_b to v_prop : Subsystem
  V : Outport
  wires:
  pos/1 -> Cross Product4/2
  pqr/1 -> Cross Product4/1
  Vb/1 -> Display2/1, Sum2/2
  i/1 -> v_b to v_prop/2(i)
  Cross Product4/1 -> Display8/1, Sum2/1
  Sum2/1 -> Display1/1, v_b to v_prop/1(V_body)
  v_b to v_prop/1(V) -> V/1

== system eVTOL_HIL/eVTOL Dynamic Model/Energy & Power/V_prop2 ==
  note: 将速度矢量投影到桨轴
  pqr : Inport
  pos : Inport  Port=2
  i : Inport  Port=3
  Vb : Inport  Port=4
  Cross Product4 : matrix_library/Cross Product
  Sum2 : Sum  Inputs=|++
  v_b to v_prop : Subsystem
  V : Outport
  wires:
  pos/1 -> Cross Product4/2
  pqr/1 -> Cross Product4/1
  Vb/1 -> Sum2/2
  i/1 -> v_b to v_prop/2(i)
  Cross Product4/1 -> Sum2/1
  Sum2/1 -> v_b to v_prop/1(V_body)
  v_b to v_prop/1(V) -> V/1

== system eVTOL_HIL/eVTOL Dynamic Model/Energy & Power/V_prop3 ==
  note: 将速度矢量投影到桨轴
  pqr : Inport
  pos : Inport  Port=2
  i : Inport  Port=3
  Va : Inport  Port=4
  Cross Product4 : matrix_library/Cross Product
  Sum2 : Sum  Inputs=|++
  v_b to v_prop : Subsystem
  V : Outport
  wires:
  pos/1 -> Cross Product4/2
  pqr/1 -> Cross Product4/1
  Va/1 -> Sum2/2
  i/1 -> v_b to v_prop/2(i)
  Cross Product4/1 -> Sum2/1
  Sum2/1 -> v_b to v_prop/1(V_body)
  v_b to v_prop/1(V) -> V/1

== system eVTOL_HIL/eVTOL Dynamic Model/Energy & Power/V_prop4 ==
  note: 将速度矢量投影到桨轴
  pqr : Inport
  pos : Inport  Port=2
  i : Inport  Port=3
  Va : Inport  Port=4
  Cross Product4 : matrix_library/Cross Product
  Sum2 : Sum  Inputs=|++
  v_b to v_prop : Subsystem
  V : Outport
  wires:
  pos/1 -> Cross Product4/2
  pqr/1 -> Cross Product4/1
  Va/1 -> Sum2/2
  i/1 -> v_b to v_prop/2(i)
  Cross Product4/1 -> Sum2/1
  Sum2/1 -> v_b to v_prop/1(V_body)
  v_b to v_prop/1(V) -> V/1

== system eVTOL_HIL/eVTOL Dynamic Model/Energy & Power/V_prop5 ==
  note: 将速度矢量投影到桨轴
  pqr : Inport
  pos : Inport  Port=2
  i : Inport  Port=3
  Va : Inport  Port=4
  Cross Product4 : matrix_library/Cross Product
  Sum2 : Sum  Inputs=|++
  v_b to v_prop : Subsystem
  V : Outport
  wires:
  pos/1 -> Cross Product4/2
  pqr/1 -> Cross Product4/1
  Va/1 -> Sum2/2
  i/1 -> v_b to v_prop/2(i)
  Cross Product4/1 -> Sum2/1
  Sum2/1 -> v_b to v_prop/1(V_body)
  v_b to v_prop/1(V) -> V/1

== system eVTOL_HIL/eVTOL Dynamic Model/Energy & Power/V_prop6 ==
  note: 将速度矢量投影到桨轴
  pqr : Inport
  pos : Inport  Port=2
  i : Inport  Port=3
  Va : Inport  Port=4
  Cross Product4 : matrix_library/Cross Product
  Sum2 : Sum  Inputs=|++
  v_b to v_prop : Subsystem
  V : Outport
  wires:
  pos/1 -> Cross Product4/2
  pqr/1 -> Cross Product4/1
  Va/1 -> Sum2/2
  i/1 -> v_b to v_prop/2(i)
  Cross Product4/1 -> Sum2/1
  Sum2/1 -> v_b to v_prop/1(V_body)
  v_b to v_prop/1(V) -> V/1

== system eVTOL_HIL/eVTOL Dynamic Model/Energy & Power/thrust_1 ==
  note: 将推力、扭矩按电机倾转角转化为向量
  note: 求桨的推力、扭矩、功率、效率
  dt : Inport
  V : Inport  Port=2
  rho : Inport  Port=3
  rpm0 : Inport  Port=4
  theta_b : Inport  Port=5
  i : Inport  Port=6
  Constant : Constant  Commented=on  Value=2.5
  Gain2 : Gain  Gain=-1
  Gain4 : Gain  Gain=pi/30
  Manual Switch : ManualSwitch  Commented=on  CurrentSetting=0
  Motor : Subsystem
  Mux1 : Mux  Inputs=2
  Mux2 : Mux  Inputs=3
  Mux3 : Mux  Inputs=2
  Mux4 : Mux  Inputs=3
  Product : Product  Inputs=*/
  "Propeller " : Subsystem
  Q_x : Fcn  Expr=-u[1]*cos(u[2])
  Q_y : Fcn  Expr=0
  Q_z : Fcn  Expr=u[1]*sin(u[2])
  Saturation : Saturate  UpperLimit=inf  LowerLimit=1
  T_x : Fcn  Expr=u[1]*cos(u[2])
  T_y : Fcn  Expr=0
  T_z : Fcn  Expr=-u[1]*sin(u[2])
  eta_plr : Outport  VectorParamsAs1DForOutWhenUnconnected=off
  Q : Outport  Port=2
  T : Outport  Port=3  VectorParamsAs1DForOutWhenUnconnected=off
  rpm : Outport  Port=4  VectorParamsAs1DForOutWhenUnconnected=off
  wires:
  Saturation/1 -> Motor/4(rpm0)
  rpm0/1 -> Saturation/1
  "Propeller "/2(T (N)) -> [T]
  dt/1 -> Motor/2(dt)
  Motor/1(rpm) -> rpm/1, Gain4/1, "Propeller "/1(rpm)
  "Propeller "/3(eta_p) -> eta_plr/1
  rho/1 -> [rho]
  "Propeller "/1(P_plr (w)) -> Motor/1(P_shaft), Product/1
  theta_b/1 -> Motor/6(theta_b), "Propeller "/4(theta_b)
  Gain4/1 -> Product/2  "omega"
  Product/1 -> Gain2/1
  T_y/1 -> Mux2/2
  Mux1/1 -> T_z/1, T_x/1, T_y/1
  T_x/1 -> Mux2/1
  i/1 -> [i]
  T_z/1 -> Mux2/3
  Mux2/1 -> T/1
  [T] -> Mux1/1
  Mux4/1 -> Q/1
  [i] -> Mux3/2
  Q_z/1 -> Mux4/3
  Q_x/1 -> Mux4/1
  Mux3/1 -> Q_z/1, Q_x/1, Q_y/1
  Q_y/1 -> Mux4/2
  [Q] -> Mux3/1
  [i] -> Mux1/2
  Gain2/1 -> [Q]
  [V] -> Motor/3(V)
  [V] -> "Propeller "/2(V)
  [rho] -> Motor/5(rho)
  [rho] -> "Propeller "/3(rho)
  Constant/1 -> Manual Switch/1
  V/1 -> [V]

== system eVTOL_HIL/eVTOL Dynamic Model/Energy & Power/thrust_2 ==
  note: 将推力、扭矩按电机倾转角转化为向量
  note: 求桨的推力、扭矩、功率、效率
  dt : Inport
  V : Inport  Port=2
  rho : Inport  Port=3
  rpm0 : Inport  Port=4
  theta_b : Inport  Port=5
  i : Inport  Port=6
  Constant : Constant  Commented=on  Value=2.5
  Gain4 : Gain  Gain=pi/30
  Manual Switch : ManualSwitch  Commented=on  CurrentSetting=0
  Motor : Subsystem
  Mux1 : Mux  Inputs=2
  Mux2 : Mux  Inputs=3
  Mux3 : Mux  Inputs=2
  Mux4 : Mux  Inputs=3
  Product : Product  Inputs=*/
  "Propeller " : Subsystem
  Q_x : Fcn  Expr=-u[1]*cos(u[2])
  Q_y : Fcn  Expr=0
  Q_z : Fcn  Expr=u[1]*sin(u[2])
  Saturation : Saturate  UpperLimit=inf  LowerLimit=1
  T_x : Fcn  Expr=u[1]*cos(u[2])
  T_y : Fcn  Expr=0
  T_z : Fcn  Expr=-u[1]*sin(u[2])
  eta_plr : Outport  VectorParamsAs1DForOutWhenUnconnected=off
  Q : Outport  Port=2
  T : Outport  Port=3  VectorParamsAs1DForOutWhenUnconnected=off
  rpm : Outport  Port=4  VectorParamsAs1DForOutWhenUnconnected=off
  wires:
  Saturation/1 -> Motor/4(rpm0)
  rpm0/1 -> Saturation/1
  "Propeller "/2(T (N)) -> [T]
  dt/1 -> Motor/2(dt)
  Motor/1(rpm) -> rpm/1, Gain4/1, "Propeller "/1(rpm)
  "Propeller "/3(eta_p) -> eta_plr/1
  rho/1 -> [rho]
  "Propeller "/1(P_plr (w)) -> Motor/1(P_shaft), Product/1
  theta_b/1 -> Motor/6(theta_b), "Propeller "/4(theta_b)
  Gain4/1 -> Product/2  "omega"
  T_y/1 -> Mux2/2
  Mux1/1 -> T_z/1, T_x/1, T_y/1
  T_x/1 -> Mux2/1
  i/1 -> [i]
  T_z/1 -> Mux2/3
  Mux2/1 -> T/1
  [T] -> Mux1/1
  Mux4/1 -> Q/1
  [i] -> Mux3/2
  Q_z/1 -> Mux4/3
  Q_x/1 -> Mux4/1
  Mux3/1 -> Q_z/1, Q_x/1, Q_y/1
  Q_y/1 -> Mux4/2
  [Q] -> Mux3/1
  [i] -> Mux1/2
  Product/1 -> [Q]
  [V] -> Motor/3(V)
  [V] -> "Propeller "/2(V)
  [rho] -> Motor/5(rho)
  [rho] -> "Propeller "/3(rho)
  Constant/1 -> Manual Switch/1
  V/1 -> [V]

== system eVTOL_HIL/eVTOL Dynamic Model/Energy & Power/thrust_3 ==
  note: 将推力、扭矩按电机倾转角转化为向量
  note: 求桨的推力、扭矩、功率、效率
  dt : Inport
  V : Inport  Port=2
  rho : Inport  Port=3
  rpm0 : Inport  Port=4
  theta_b : Inport  Port=5
  i : Inport  Port=6
  Constant : Constant  Commented=on  Value=2.5
  Gain4 : Gain  Gain=pi/30
  Manual Switch : ManualSwitch  Commented=on  CurrentSetting=0
  Motor : Subsystem
  Mux1 : Mux  Inputs=2
  Mux2 : Mux  Inputs=3
  Mux3 : Mux  Inputs=2
  Mux4 : Mux  Inputs=3
  Product : Product  Inputs=*/
  "Propeller " : Subsystem
  Q_x : Fcn  Expr=-u[1]*cos(u[2])
  Q_y : Fcn  Expr=0
  Q_z : Fcn  Expr=u[1]*sin(u[2])
  Saturation : Saturate  UpperLimit=inf  LowerLimit=1
  T_x : Fcn  Expr=u[1]*cos(u[2])
  T_y : Fcn  Expr=0
  T_z : Fcn  Expr=-u[1]*sin(u[2])
  eta_plr : Outport  VectorParamsAs1DForOutWhenUnconnected=off
  Q : Outport  Port=2
  T : Outport  Port=3  VectorParamsAs1DForOutWhenUnconnected=off
  rpm : Outport  Port=4  VectorParamsAs1DForOutWhenUnconnected=off
  wires:
  Saturation/1 -> Motor/4(rpm0)
  rpm0/1 -> Saturation/1
  "Propeller "/2(T (N)) -> [T]
  dt/1 -> Motor/2(dt)
  Motor/1(rpm) -> rpm/1, Gain4/1, "Propeller "/1(rpm)
  "Propeller "/3(eta_p) -> eta_plr/1
  rho/1 -> [rho]
  "Propeller "/1(P_plr (w)) -> Motor/1(P_shaft), Product/1
  theta_b/1 -> Motor/6(theta_b), "Propeller "/4(theta_b)
  Gain4/1 -> Product/2  "omega"
  T_y/1 -> Mux2/2
  Mux1/1 -> T_z/1, T_x/1, T_y/1
  T_x/1 -> Mux2/1
  i/1 -> [i]
  T_z/1 -> Mux2/3
  Mux2/1 -> T/1
  [T] -> Mux1/1
  Mux4/1 -> Q/1
  [i] -> Mux3/2
  Q_z/1 -> Mux4/3
  Q_x/1 -> Mux4/1
  Mux3/1 -> Q_z/1, Q_x/1, Q_y/1
  Q_y/1 -> Mux4/2
  [Q] -> Mux3/1
  [i] -> Mux1/2
  Product/1 -> [Q]
  [V] -> Motor/3(V)
  [V] -> "Propeller "/2(V)
  [rho] -> Motor/5(rho)
  [rho] -> "Propeller "/3(rho)
  Constant/1 -> Manual Switch/1
  V/1 -> [V]

== system eVTOL_HIL/eVTOL Dynamic Model/Energy & Power/thrust_4 ==
  note: 将推力、扭矩按电机倾转角转化为向量
  note: 求桨的推力、扭矩、功率、效率
  dt : Inport
  V : Inport  Port=2
  rho : Inport  Port=3
  rpm0 : Inport  Port=4
  theta_b : Inport  Port=5
  i : Inport  Port=6
  Constant : Constant  Commented=on  Value=2.5
  Gain2 : Gain  Gain=-1
  Gain4 : Gain  Gain=pi/30
  Manual Switch : ManualSwitch  Commented=on  CurrentSetting=0
  Motor : Subsystem
  Mux1 : Mux  Inputs=2
  Mux2 : Mux  Inputs=3
  Mux3 : Mux  Inputs=2
  Mux4 : Mux  Inputs=3
  Product : Product  Inputs=*/
  "Propeller " : Subsystem
  Q_x : Fcn  Expr=-u[1]*cos(u[2])
  Q_y : Fcn  Expr=0
  Q_z : Fcn  Expr=u[1]*sin(u[2])
  Saturation : Saturate  UpperLimit=inf  LowerLimit=1
  T_x : Fcn  Expr=u[1]*cos(u[2])
  T_y : Fcn  Expr=0
  T_z : Fcn  Expr=-u[1]*sin(u[2])
  eta_plr : Outport  VectorParamsAs1DForOutWhenUnconnected=off
  Q : Outport  Port=2
  T : Outport  Port=3  VectorParamsAs1DForOutWhenUnconnected=off
  rpm : Outport  Port=4  VectorParamsAs1DForOutWhenUnconnected=off
  wires:
  Saturation/1 -> Motor/4(rpm0)
  rpm0/1 -> Saturation/1
  "Propeller "/2(T (N)) -> [T]
  dt/1 -> Motor/2(dt)
  Motor/1(rpm) -> rpm/1, Gain4/1, "Propeller "/1(rpm)
  "Propeller "/3(eta_p) -> eta_plr/1
  rho/1 -> [rho]
  "Propeller "/1(P_plr (w)) -> Motor/1(P_shaft), Product/1
  theta_b/1 -> Motor/6(theta_b), "Propeller "/4(theta_b)
  Gain4/1 -> Product/2  "omega"
  T_y/1 -> Mux2/2
  Mux1/1 -> T_z/1, T_x/1, T_y/1
  T_x/1 -> Mux2/1
  i/1 -> [i]
  T_z/1 -> Mux2/3
  Mux2/1 -> T/1
  [T] -> Mux1/1
  Mux4/1 -> Q/1
  [i] -> Mux3/2
  Q_z/1 -> Mux4/3
  Q_x/1 -> Mux4/1
  Mux3/1 -> Q_z/1, Q_x/1, Q_y/1
  Q_y/1 -> Mux4/2
  [Q] -> Mux3/1
  [i] -> Mux1/2
  Product/1 -> Gain2/1
  [V] -> Motor/3(V)
  [V] -> "Propeller "/2(V)
  [rho] -> Motor/5(rho)
  [rho] -> "Propeller "/3(rho)
  Gain2/1 -> [Q]
  Constant/1 -> Manual Switch/1
  V/1 -> [V]

== system eVTOL_HIL/eVTOL Dynamic Model/Energy & Power/thrust_5 ==
  note: 将推力、扭矩按电机倾转角转化为向量
  note: 求桨的推力、扭矩、功率、效率
  dt : Inport
  V : Inport  Port=2
  rho : Inport  Port=3
  rpm0 : Inport  Port=4
  theta_b : Inport  Port=5
  i : Inport  Port=6
  Constant : Constant  Commented=on  Value=2.5
  Gain2 : Gain  Gain=-1
  Gain4 : Gain  Gain=pi/30
  Manual Switch : ManualSwitch  Commented=on  CurrentSetting=0
  Motor : Subsystem
  Mux1 : Mux  Inputs=2
  Mux2 : Mux  Inputs=3
  Mux3 : Mux  Inputs=2
  Mux4 : Mux  Inputs=3
  Product : Product  Inputs=*/
  "Propeller " : Subsystem
  Q_x : Fcn  Expr=-u[1]*cos(u[2])
  Q_y : Fcn  Expr=0
  Q_z : Fcn  Expr=u[1]*sin(u[2])
  Saturation : Saturate  UpperLimit=inf  LowerLimit=1
  T_x : Fcn  Expr=u[1]*cos(u[2])
  T_y : Fcn  Expr=0
  T_z : Fcn  Expr=-u[1]*sin(u[2])
  eta_plr : Outport  VectorParamsAs1DForOutWhenUnconnected=off
  Q : Outport  Port=2
  T : Outport  Port=3  VectorParamsAs1DForOutWhenUnconnected=off
  rpm : Outport  Port=4  VectorParamsAs1DForOutWhenUnconnected=off
  wires:
  Saturation/1 -> Motor/4(rpm0)
  rpm0/1 -> Saturation/1
  "Propeller "/2(T (N)) -> [T]
  dt/1 -> Motor/2(dt)
  Motor/1(rpm) -> rpm/1, Gain4/1, "Propeller "/1(rpm)
  "Propeller "/3(eta_p) -> eta_plr/1
  rho/1 -> [rho]
  "Propeller "/1(P_plr (w)) -> Motor/1(P_shaft), Product/1
  theta_b/1 -> Motor/6(theta_b), "Propeller "/4(theta_b)
  Gain4/1 -> Product/2  "omega"
  T_y/1 -> Mux2/2
  Mux1/1 -> T_z/1, T_x/1, T_y/1
  T_x/1 -> Mux2/1
  i/1 -> [i]
  T_z/1 -> Mux2/3
  Mux2/1 -> T/1
  [T] -> Mux1/1
  Mux4/1 -> Q/1
  [i] -> Mux3/2
  Q_z/1 -> Mux4/3
  Q_x/1 -> Mux4/1
  Mux3/1 -> Q_z/1, Q_x/1, Q_y/1
  Q_y/1 -> Mux4/2
  [Q] -> Mux3/1
  [i] -> Mux1/2
  Product/1 -> Gain2/1
  [V] -> Motor/3(V)
  [V] -> "Propeller "/2(V)
  [rho] -> Motor/5(rho)
  [rho] -> "Propeller "/3(rho)
  Gain2/1 -> [Q]
  Constant/1 -> Manual Switch/1
  V/1 -> [V]

== system eVTOL_HIL/eVTOL Dynamic Model/Energy & Power/thrust_6 ==
  note: 将推力、扭矩按电机倾转角转化为向量
  note: 求桨的推力、扭矩、功率、效率
  dt : Inport
  V : Inport  Port=2
  rho : Inport  Port=3
  rpm0 : Inport  Port=4
  theta_b : Inport  Port=5
  i : Inport  Port=6
  Constant : Constant  Commented=on  Value=2.5
  Gain4 : Gain  Gain=pi/30
  Manual Switch : ManualSwitch  Commented=on  CurrentSetting=0
  Motor : Subsystem
  Mux1 : Mux  Inputs=2
  Mux2 : Mux  Inputs=3
  Mux3 : Mux  Inputs=2
  Mux4 : Mux  Inputs=3
  Product : Product  Inputs=*/
  "Propeller " : Subsystem
  Q_x : Fcn  Expr=-u[1]*cos(u[2])
  Q_y : Fcn  Expr=0
  Q_z : Fcn  Expr=u[1]*sin(u[2])
  Saturation : Saturate  UpperLimit=inf  LowerLimit=1
  T_x : Fcn  Expr=u[1]*cos(u[2])
  T_y : Fcn  Expr=0
  T_z : Fcn  Expr=-u[1]*sin(u[2])
  eta_plr : Outport  VectorParamsAs1DForOutWhenUnconnected=off
  Q : Outport  Port=2
  T : Outport  Port=3  VectorParamsAs1DForOutWhenUnconnected=off
  rpm : Outport  Port=4  VectorParamsAs1DForOutWhenUnconnected=off
  wires:
  Saturation/1 -> Motor/4(rpm0)
  rpm0/1 -> Saturation/1
  "Propeller "/2(T (N)) -> [T]
  dt/1 -> Motor/2(dt)
  Motor/1(rpm) -> rpm/1, Gain4/1, "Propeller "/1(rpm)
  "Propeller "/3(eta_p) -> eta_plr/1
  rho/1 -> [rho]
  "Propeller "/1(P_plr (w)) -> Motor/1(P_shaft), Product/1
  theta_b/1 -> Motor/6(theta_b), "Propeller "/4(theta_b)
  Gain4/1 -> Product/2  "omega"
  T_y/1 -> Mux2/2
  Mux1/1 -> T_z/1, T_x/1, T_y/1
  T_x/1 -> Mux2/1
  i/1 -> [i]
  T_z/1 -> Mux2/3
  Mux2/1 -> T/1
  [T] -> Mux1/1
  Mux4/1 -> Q/1
  [i] -> Mux3/2
  Q_z/1 -> Mux4/3
  Q_x/1 -> Mux4/1
  Mux3/1 -> Q_z/1, Q_x/1, Q_y/1
  Q_y/1 -> Mux4/2
  [Q] -> Mux3/1
  [i] -> Mux1/2
  [V] -> Motor/3(V)
  [V] -> "Propeller "/2(V)
  [rho] -> Motor/5(rho)
  [rho] -> "Propeller "/3(rho)
  Product/1 -> [Q]
  Constant/1 -> Manual Switch/1
  V/1 -> [V]

== system eVTOL_HIL/eVTOL Dynamic Model/Environment/Terrain ==
  Xe : Inport
  Terminator : Terminator
  hground_value : Constant  OutDataTypeStr=single
  hground : Outport  VectorParamsAs1DForOutWhenUnconnected=off
  wires:
  Xe/1 -> Terminator/1
  hground_value/1 -> hground/1  "hground"
